simulink model "bintang_Command_Windows"  (R2023a)
settings: Solver=VariableStepAuto  StartTime=0.0  StopTime=10.0  RelTol=1e-3
values from neighbouring files (symbols this model uses):
  Ts1 = 0.2    [Command windows.mat]    (also in Zero-order.mat)
  Ts2 = 0.5    [Command windows.mat]    (also in Zero-order.mat)
settings Model: Creator=Lenovo  LastModifiedBy=Lenovo

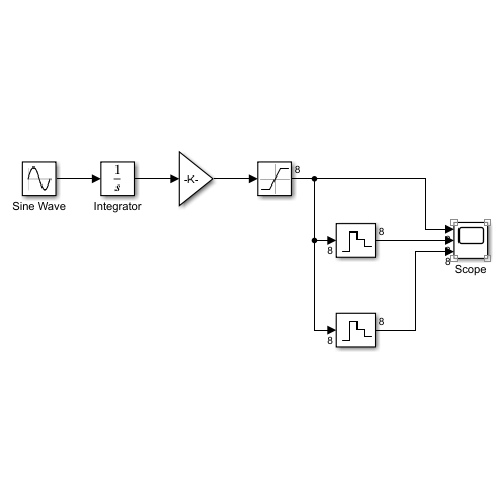
[thumbnail: Simulink's stored preview of the top-level diagram]
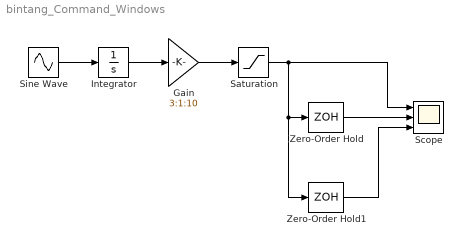
== system bintang_Command_Windows ==
  Gain : Gain  Gain=3:1:10
  Integrator : Integrator
  Saturation : Saturate  UpperLimit=rand(8,1)*10  LowerLimit=rand(8,1)*.10
  Scope : Scope  NumInputPorts=3
  Sine Wave : Sin  Amplitude=0.5  SampleTime=0
  Zero-Order Hold : ZeroOrderHold  SampleTime=Ts1
  Zero-Order Hold1 : ZeroOrderHold  SampleTime=Ts2
  wires:
  Gain/1 -> Saturation/1
  Integrator/1 -> Gain/1
  Sine Wave/1 -> Integrator/1
  Saturation/1 -> Zero-Order Hold1/1, Zero-Order Hold/1, Scope/1
  Zero-Order Hold/1 -> Scope/2
  Zero-Order Hold1/1 -> Scope/3
